simulink library "carnot"  (R2013b)
settings: Solver=ode45  StartTime=0.0  StopTime=10.0  RelTol=1e-3
undefined symbols (not defined in the file or in its folder): A, acol, Ahabit, Awin, Azimuth_Angle, AziWin, B, C, c1, c4, capc, caph, CarnotCallbacks_Density, CarnotCallbacks_Enthalpy, CarnotCallbacks_Enthalpy2Temperature, CarnotCallbacks_Entropy, CarnotCallbacks_Evaporation_Enthalpy, CarnotCallbacks_GlobalMessageLevel, CarnotCallbacks_Grashof, CarnotCallbacks_Heat_Capacity, CarnotCallbacks_Kinematic_Viscosity, CarnotCallbacks_Prandtl, CarnotCallbacks_Saturation_Property, CarnotCallbacks_Saturation_Temperature, CarnotCallbacks_Saturation_Value_Water, CarnotCallbacks_Specific_Volume, CarnotCallbacks_Thermal_Conductivity, CarnotCallbacks_Vapour_Content, CarnotCallbacks_Vapour_Pressure, con, cond, d, Dd, density, dfin, dia, DiameterLastPiece, DPConstant, dpipe, DPLinear, DPQuadratic, emission_out, fluid, FluidMix, FluidType, FPC, frame, g, GeodeticHeight, Gwin, heat_capacity, hgt, HP, Hroom, ID, inlet, K, l, lin, lpipe ... (+29)
undefined symbols (not defined in the file): c2, c3, c5, c6, cwall, dactive, height, mc, mID, rho, tau, UAneighbour, UAwall, uloss
libraries: carnot x333, simulink x25, simulink_extras x7
(part 8 of 16)

== system carnot/Storage/Thermal ==
  Ground_Storage : Subsystem  mask(ground storage){xs=10, ys=10, zs=5, ground=clay (humid), fill=clay (humid), dp=0.1, kp=0.001, zp=1, np=20, t0=20, refine=1, mpts=5}
      mask prompts: xs "extension perpendicular to pipes [m]"; ys "extension parallel to pipes [m]"; zs "depth of storage [m]"; fill "filling"; dp "diameter of pipe [m]"; kp "roughness of pipe [m]"; zp "depth of pipe [m]"; np "number of pipes"; t0 "initial temperature [degree centigrade]"; refine "refine factor"; mpts "number of measurement points"
      mask help:
      | Three-dimensional ground storage model.
      | Look under mask to change the surface model.
      mask init:
      | xs = max(xs, 0.001);
      | ys = max(ys, 0.001);
      | zp = max(zp, 0.001);
      | zs = max(zs, zp);
      | np = max(0, np);
      | dp = max(dp, 0.001);
      | kp = max(kp, 0.001);
      | cond=[0.7 1.88 1.45 2.9 1.28];
      | lg = cond(ground);
      | cap = [1382400 1798200 2410560  2864160 1933800];
      | cg = cap(ground);
      | lf = cond(fill);
      | cf = cap(fill);
      mask Help: web(fullfile(path_carnot('help'),'Ground_Storage.html'),'-helpbrowser')
      mask TypeOptions ground: sand (dry) | sand (saturated with water) | clay (humid) | clay (saturated with water)
      mask TypeOptions fill: sand (dry) | sand (saturated with water) | clay (humid) | clay (saturated with water) | concrete
      mask TypeOptions refine: 1 | 2 | 3 | 4 | 6 | 8 | 10 | 16 | 24 | 32
      mask Display: plot(0,0,100,100,[30,60,70,40,30],[70,70,80,80,70],[68,59,56,59,56,52,48,51,48,44,40,44,41,32],[83,72,72,78,78,72,72,78,78,72,72,78,78,67],[61,58,44,31,30],[69,60,56,60,67],[62,60,52,37,29,29],[68,56,47,48,57,67],[64,67,67,65,57,44,32,27,28],[71,62,53,43,35,35,40,54,66])
  Storage_Ports : Subsystem
      mask Display: plot(0,0,100,100,[10,10,40,40,10],[10,40,40,10,10],[50,70,90,50],[30,65,30,30],[20,10,10,20,30,40,40,30,20],[50,60,70,80,80,70,60,50,50])
  Storage_Type_1 : Subsystem  mask(Multiport Storage){uloss=1, ubot=1, utop=1, cond=1, t0=[10:5:55], volume=0.3, dia=0.5, pos=standing cylinder, nconnect=2, nodes=10, mpoints=10}
      mask prompts: uloss "Heat loss coefficient cylinder wall in W/(m²K)"; ubot "Heat loss coefficient bottom in W/(m²K)"; utop "Heat loss coefficient top cover in W/(m²K)"; cond "Effective vertical conductivity in W/(m*K)"; t0 "Initial temperature (vector or scalar) in °C"; volume "Volume in m³"; dia "Diameter in m"; pos "Position"; nconnect "Number of connections"; nodes "Number of nodes"; mpoints "Number of measurement points"
      mask help:
      | The volmue of the cylindrical storage is divided in a number "nodes" of horizontal slices (1xN-node model). For each node the energy balance equation is solved.
      | Look under mask to set the ports types and properties.
      mask init:
      | [standing, dh, height, mpts, tini] ...
      |     = CarnotCallbacks_StorageTypeN(pos, volume, dia, nodes, mpoints, t0);
      mask Help: web(fullfile(path_carnot('help'),'Storage_Type_N.html'),'-helpbrowser')
      mask TypeOptions pos: lying cylinder | standing cylinder
      mask Display: plot(10,10,90,100,[40,40,45,55,60,60,55,45,40],[84,36,30,30,36,84,90,90,84],[40,35],[77,77],[64,60],[77,77],[40,35],[42,42],[64,60],[42,42])
  Storage_Type_1_CONF : Subsystem  mask(Buffer Storage with 2 connections){parameterfile=default_Storage, tini=[10:5:55]}
      mask prompts: parameterfile "Storage parameter set"; tini "initial temperature (vector or scalar) in °C"
      mask help: Predefinded storage with 2 direct ports (for example a buffer storage tank).
      mask init:
      | % callback to set parameters of model
      | CarnotCallbacks_StorageConf(1,parameterfile);
      mask Help: web(fullfile(path_carnot('help'),'Storage_Type_N.html'),'-helpbrowser')
      mask TypeOptions parameterfile: default_Storage
      mask Display:
      | % user defined picture file
      | picfile = fullfile(path_carnot('intlibsl'), ...
      |     'Storage','Thermal','Storage_Type_1_CONF','parameter_set', ...
      |     'Storage_Type_1_CONF.jpg');
      | 
      | % show public picture
      | plot([40,40,45,55,60,60,55,45,40]/100,[84,36,30,30,36,84,90,90,84]/100, ...
      |     [40,35]/100,[77,77]/100,[64,60]/100,[77,77]/100,[40,35]/100,[42,42]/100, ...
      |     [64,60]/100,[42,42]/100)
      | 
      | % show internal picture if defined
      | if ~BlockIsInCarnotLibrary    % if not located in library any more
      |     if exist(picfile)
      |         image(imread(picfile), [0.3, 0, 0.5, 1])
      |         set_param(gcb, 'BackgroundColor', 'White')
      |     end
      | end
  Storage_Type_2 : Subsystem  mask(Multiport Storage){uloss=1, ubot=1, utop=1, cond=1, t0=[10:5:55], volume=0.3, dia=0.5, pos=standing cylinder, nconnect=2, nodes=10, mpoints=10}
      mask prompts: uloss "Heat loss coefficient cylinder wall in W/(m²K)"; ubot "Heat loss coefficient bottom in W/(m²K)"; utop "Heat loss coefficient top cover in W/(m²K)"; cond "Effective vertical conductivity in W/(m*K)"; t0 "Initial temperature (vector or scalar) in °C"; volume "Volume in m³"; dia "Diameter in m"; pos "Position"; nconnect "Number of connections"; nodes "Number of nodes"; mpoints "Number of measurement points"
      mask help:
      | The volmue of the cylindrical storage is divided in a number "nodes" of horizontal slices (1xN-node model). For each node the energy balance equation is solved.
      | Look under mask to set the ports types and properties.
      mask init:
      | [standing, dh, height, mpts, tini] ...
      |     = CarnotCallbacks_StorageTypeN(pos, volume, dia, nodes, mpoints, t0);
      mask Help: web(fullfile(path_carnot('help'),'Storage_Type_N.html'),'-helpbrowser')
      mask TypeOptions pos: lying cylinder | standing cylinder
      mask Display: plot(10,20,80,100,[36,36,40,50,54,54,50,40,36],[90,50,45,45,50,90,93,93,90],[36,51,44,51,36],[50,50,55,60,60])
  Storage_Type_2_CONF : Subsystem  mask(Storage with 1 heat exchanger and 1 direct port){parameterfile=default_Storage, tini=[10:5:55]}
      mask prompts: parameterfile "Storage parameter set"; tini "initial temperature (vector or scalar) in °C"
      mask help: Predefinded storage with 1 heat exchanger and 1 direct port (for example a dhw cylinder).
      mask init:
      | % callback to set parameters of model
      | CarnotCallbacks_StorageConf(2,parameterfile);
      mask Help: web(fullfile(path_carnot('help'),'Storage_Type_N.html'),'-helpbrowser')
      mask TypeOptions parameterfile: default_Storage
      mask Display:
      | % user defined picture file
      | picfile = fullfile(path_carnot('intlibsl'), ...
      |         'Storage','Thermal','Storage_Type_2_CONF','parameter_set', ...
      |         'Storage_Type_2_CONF.jpg');
      | 
      | % show public picture
      | plot(0.1,0.2,0.80,1,[36,36,40,50,54,54,50,40,36]/100,...
      |     [90,50,45,45,50,90,93,93,90]/100,[36,51,44,51,36]/100,...
      |     [50,50,55,60,60]/100)
      | 
      | % show internal picture if defined
      | if  ~BlockIsInCarnotLibrary       % if not located in library
      |     if exist(picfile)
      |         image(imread(picfile), [0.3, 0, 0.5, 1])
      |         set_param(gcb, 'BackgroundColor', 'White')
      |     end
      | end
  Storage_Type_3 : Subsystem  mask(Multiport Storage){uloss=1, ubot=1, utop=1, cond=1, t0=[10:5:55], volume=0.3, dia=0.5, pos=standing cylinder, nconnect=3, nodes=10, mpoints=10}
      mask prompts: uloss "Heat loss coefficient cylinder wall in W/(m²K)"; ubot "Heat loss coefficient bottom in W/(m²K)"; utop "Heat loss coefficient top cover in W/(m²K)"; cond "Effective (wall and fluid) vertical conductivity in W/(m*K)"; t0 "Initial temperature (vector or scalar) in °C"; volume "Volume in m³"; dia "Diameter in m"; pos "Position"; nconnect "Number of connections"; nodes "Number of nodes"; mpoints "Number of measurement points"
      mask help:
      | The volmue of the cylindrical storage is divided in a number "nodes" of horizontal slices (1xN-node model). For each node the energy balance equation is solved.
      | Look under mask to set the ports types and properties.
      mask init:
      | [standing, dh, height, mpts, tini] ...
      |     = CarnotCallbacks_StorageTypeN(pos, volume, dia, nodes, mpoints, t0);
      mask Help: web(fullfile(path_carnot('help'),'Storage_Type_N.html'),'-helpbrowser')
      mask TypeOptions pos: lying cylinder | standing cylinder
      mask Display: plot(10,20,80,100,[36,36,40,50,54,54,50,40,36],[90,50,45,45,50,90,93,93,90],[36,51,40,51,36],[77,77,81,85,85],[36,51,44,51,36],[50,50,55,60,60])
  Storage_Type_3_CONF : Subsystem  mask(Storage with 2 heat exchangers and 1 direct port){parameterfile=default_Storage, tini=[10:5:55]}
      mask prompts: parameterfile "Storage parameter set"; tini "initial temperature (vector or scalar) in °C"
      mask help: Predefinded storage with 2 heat exchangers and 1 direct port (for example a bivalent dhw cylinder).
      mask init:
      | % callback to set parameters of model
      | CarnotCallbacks_StorageConf(3,parameterfile);
      mask Help: web(fullfile(path_carnot('help'),'Storage_Type_N.html'),'-helpbrowser')
      mask TypeOptions parameterfile: default_Storage
      mask Display:
      | % user defined picture file
      | picfile = fullfile(path_carnot('intlibsl'), ...
      |         'Storage','Thermal','Storage_Type_3_CONF','parameter_set', ...
      |         'Storage_Type_3_CONF.jpg');
      | 
      | % show public picture
      | plot([36,36,40,50,54,54,50,40,36]/100,[90,50,45,45,50,90,93,93,90]/100, ...
      |     [36,51,40,51,36]/100,[77,77,81,85,85]/100,[36,51,44,51,36]/100, ...
      |     [50,50,55,60,60]/100)
      | 
      | % show internal picture if defined
      | if  ~BlockIsInCarnotLibrary       % if not located in library
      |     if exist(picfile)
      |         image(imread(picfile), [0.25, 0, 0.45, 1])
      |         set_param(gcb, 'BackgroundColor', 'White')
      |     end
      | end
  Storage_Type_4 : Subsystem  mask(Multiport Storage){uloss=0.74, ubot=1.37, utop=0.74, cond=0.62, t0=[10:5:55], volume=0.75, dia=0.79, pos=standing cylinder, nconnect=4, nodes=50, mpoints=50}
      mask prompts: uloss "Heat loss coefficient cylinder wall in W/(m²K)"; ubot "Heat loss coefficient bottom in W/(m²K)"; utop "Heat loss coefficient top cover in W/(m²K)"; cond "Effective (wall and fluid) vertical conductivity in W/(m*K)"; t0 "Initial temperature (vector or scalar) in °C"; volume "Volume in m³"; dia "Diameter in m"; pos "Position"; nconnect "Number of connections"; nodes "Number of nodes"; mpoints "Number of measurement points"
      mask help:
      | The volmue of the cylindrical storage is divided in a number "nodes" of horizontal slices (1xN-node model). For each node the energy balance equation is solved.
      | Look under mask to set the ports types and properties.
      mask init:
      | [standing, dh, height, mpts, tini] ...
      |     = CarnotCallbacks_StorageTypeN(pos, volume, dia, nodes, mpoints, t0);
      mask Help: web(fullfile(path_carnot('help'),'Storage_Type_N.html'),'-helpbrowser')
      mask TypeOptions pos: lying cylinder | standing cylinder
      mask Display: plot(5,10,85,110,[36,36,40,50,54,54,50,40,36],[90,50,45,45,50,90,93,93,90],[36,51,40,51,36],[50,50,68,85,85],[36,51,44,51,36],[54,54,56,58,58])
  Storage_Type_4_CONF : Subsystem  mask(Combi-storage for hot water production and heating){parameterfile=Default_Storage, tini=[10:5:55]}
      mask prompts: parameterfile "Storage parameter set"; tini "initial temperature (vector or scalar) in °C"
      mask help: Predefinded combi-storage for hot water production and heating configurated to preheat the return of the backup heater.
      mask init:
      | % callback to set parameters of model
      | CarnotCallbacks_StorageConf(4,parameterfile);
      mask Help: web(fullfile(path_carnot('help'),'Storage_Type_N.html'),'-helpbrowser')
      mask TypeOptions parameterfile: Default_Storage
      mask Display:
      | % user defined picture file
      | picfile = fullfile(path_carnot('intlibsl'), ...
      |         'Storage','Thermal','Storage_Type_4_CONF','parameter_set', ...
      |         'Storage_Type_4_CONF.jpg');
      | 
      | % show public picture
      | plot([36,36,40,50,54,54,50,40,36]/100,[90,50,45,45,50,90,93,93,90]/100, ...
      |     [36,51,40,51,36]/100,[50,50,68,85,85]/100,[36,51,44,51,36]/100, ...
      |     [54,54,56,58,58]/100)
      | 
      | % show internal picture if defined
      | if  ~BlockIsInCarnotLibrary       % if not located in library
      |     if exist(picfile)
      |         image(imread(picfile), [0.3, 0, 0.45, 1])
      |         set_param(gcb, 'BackgroundColor', 'White')
      |     end
      | end
  Storage_Type_5 : Subsystem  mask(Multiport Storage){uloss=0.74, ubot=1.37, utop=0.74, cond=0.62, t0=[10:5:55], volume=0.75, dia=0.79, pos=standing cylinder, nconnect=5, nodes=50, mpoints=50}
      mask prompts: uloss "Heat loss coefficient cylinder wall in W/(m²K)"; ubot "Heat loss coefficient bottom in W/(m²K)"; utop "Heat loss coefficient top cover in W/(m²K)"; cond "Effective (wall and fluid) vertical conductivity in W/(m*K)"; t0 "Initial temperature (vector or scalar) in °C"; volume "Volume in m³"; dia "Diameter in m"; pos "Position"; nconnect "Number of connections"; nodes "Number of nodes"; mpoints "Number of measurement points"
      mask help:
      | The volmue of the cylindrical storage is divided in a number "nodes" of horizontal slices (1xN-node model). For each node the energy balance equation is solved.
      | Look under mask to set the ports types and properties.
      mask init:
      | [standing, dh, height, mpts, tini] ...
      |     = CarnotCallbacks_StorageTypeN(pos, volume, dia, nodes, mpoints, t0);
      mask Help: web(fullfile(path_carnot('help'),'Storage_Type_N.html'),'-helpbrowser')
      mask TypeOptions pos: lying cylinder | standing cylinder
      mask Display: plot(5,10,85,110,[36,36,40,50,54,54,50,40,36],[90,50,45,45,50,90,93,93,90],[36,51,40,51,36],[50,50,68,85,85],[36,51,44,51,36],[54,54,56,58,58])
  Storage_Type_5_CONF : Subsystem  mask(Combi-storage for hot water production and heating){parameterfile=Default_Storage, tini=[10:5:55]}
      mask prompts: parameterfile "Storage parameter set"; tini "initial temperature (vector or scalar) in °C"
      mask help: Predefinded combi-storage for hot water production and heating configurated for parallel buffer operation of the backup heater.
      mask init:
      | % callback to set parameters of model
      | CarnotCallbacks_StorageConf(5,parameterfile);
      mask Help: web(fullfile(path_carnot('help'),'Storage_Type_N.html'),'-helpbrowser')
      mask TypeOptions parameterfile: Default_Storage
      mask Display:
      | % user defined picture file
      | picfile = fullfile(path_carnot('intlibsl'), ...
      |         'Storage','Thermal','Storage_Type_5_CONF','parameter_set', ...
      |         'Storage_Type_5_CONF.jpg');
      | 
      | % show public picture
      | plot([36,36,40,50,54,54,50,40,36]/100,[90,50,45,45,50,90,93,93,90]/100, ...
      |     [36,51,40,51,36]/100,[50,50,68,85,85]/100,[36,51,44,51,36]/100, ...
      |     [54,54,56,58,58]/100)
      | 
      | % show internal picture if defined
      | if  ~BlockIsInCarnotLibrary       % if not located in library
      |     if exist(picfile)
      |         image(imread(picfile), [0.3, 0, 0.45, 1])
      |         set_param(gcb, 'BackgroundColor', 'White')
      |     end
      | end
  detailed_storage_models : Subsystem
      mask Display: plot(0,0,100,100,[10,10,40,40,10],[10,40,40,10,10],[50,70,90,50],[30,65,30,30],[20,10,10,20,30,40,40,30,20],[50,60,70,80,80,70,60,50,50])
  surface_models : Subsystem
      mask Display: plot(0,0,100,100,[10,10,40,40,10],[10,40,40,10,10],[50,70,90,50],[30,65,30,30],[20,10,10,20,30,40,40,30,20],[50,60,70,80,80,70,60,50,50])

== system carnot/Toolbox/Average ==
  input : Inport
  time : Inport  Port=2
  enable : Inport  Port=3
  Demux1 : Demux  Outputs=[-1 1 1]
  Mux : Mux  Inputs=3
  S-Function3 : S-Function  FunctionName=average  Parameters=delta_t offset_flag enable_flag  EnableBusSupport=off
  average : Outport
  output time : Outport  Port=2
  pulse : Outport  Port=3
  wires:
  Mux/1 -> S-Function3/1
  S-Function3/1 -> Demux1/1
  input/1 -> Mux/1
  time/1 -> Mux/2
  enable/1 -> Mux/3
  Demux1/1 -> average/1
  Demux1/2 -> output time/1
  Demux1/3 -> pulse/1

== system carnot/Toolbox/Economy_Ecology ==
  note: mass of fuel in kg
  note: thermal energy in J
  note: electric energy in J
  note: fuel costs
  note: mass of produced H2O
  note: mass of produced CO2
  note: mass of produced O2
  note: mass of produced SO2
  note: mass of produced N2
  note: mass of produced NOx
  note: mass of produced CO
  note: mass of produced CxHy
  eco : Inport
  Count_Working_Time : carnot/Toolbox/Count_Working_Time
  Demux1 : Demux  Outputs=12
  Display : Display
  Integrator : Integrator
  Mux : Mux  Inputs=12
  Mux1 : Mux  Inputs=2
  Selector : Selector  InputPortWidth=19  IndexOptions=Index vector (dialog)  Indices=[3 5:15]  OutputSizes=1
  Selector1 : Selector  InputPortWidth=12  IndexOptions=Index vector (dialog)  Indices=[1]  OutputSizes=1
  Terminator : Terminator
  Terminator1 : Terminator
  Terminator2 : Terminator
  To Workspace : ToWorkspace  VariableName=input_annual_costs  SampleTime=-1
      settings: MaxDataPoints=1
  wires:
  Count_Working_Time/3 -> Terminator2/1
  Count_Working_Time/2 -> Terminator1/1
  Count_Working_Time/1 -> Terminator/1
  Count_Working_Time/4 -> Mux1/2  "Run time"
  Demux1/4 -> Mux1/1, Mux/4  "costs"
  Demux1/1 -> Mux/1  "m_fuel"
  Selector1/1 -> Count_Working_Time/1
  Selector/1 -> Selector1/1, Integrator/1
  Mux1/1 -> To Workspace/1
  Mux/1 -> Display/1
  Demux1/3 -> Mux/3  "E_electric"
  Demux1/2 -> Mux/2  "Qtherm"
  Demux1/10 -> Mux/10  "NOx"
  Demux1/11 -> Mux/11  "CO"
  Demux1/12 -> Mux/12  "CxHy"
  Demux1/9 -> Mux/9  "N2"
  Demux1/6 -> Mux/6  "CO2"
  Integrator/1 -> Demux1/1
  eco/1 -> Selector/1
  Demux1/7 -> Mux/7  "O2"
  Demux1/5 -> Mux/5  "H20"
  Demux1/8 -> Mux/8  "SO2"

== system carnot/Toolbox/GlobalMessageLevel ==

== system carnot/Toolbox/RealDate ==
  Ground : Ground
  S-Function3 : S-Function  FunctionName=systemdate  Parameters=form  EnableBusSupport=off
  date : Outport
  wires:
  S-Function3/1 -> date/1
  Ground/1 -> S-Function3/1

== system carnot/Toolbox/RealTime ==
  Ground : Ground
  S-Function3 : S-Function  FunctionName=systemtime  EnableBusSupport=off
  time : Outport
  wires:
  S-Function3/1 -> time/1
  Ground/1 -> S-Function3/1

== system carnot/Toolbox/RealTimePulse ==
  In : Inport
  S-Function : S-Function  FunctionName=monoflop_realtime  Parameters=time typ  EnableBusSupport=off
  Out : Outport
  wires:
  In/1 -> S-Function/1
  S-Function/1 -> Out/1

== system carnot/Toolbox/SystemPulse ==
  enable pulse : Inport
  Mux : Mux  Inputs=2
  S-Function3 : S-Function  FunctionName=systempulse  Parameters=datecheck enable_flag  EnableBusSupport=off
  position6 : Constant  Value=[date period pulsewidth]
  pulse : Outport
  wires:
  Mux/1 -> S-Function3/1
  enable pulse/1 -> Mux/2
  S-Function3/1 -> pulse/1
  position6/1 -> Mux/1

== system carnot/Toolbox/THB2THV ==
  THB : Inport  OutDataTypeStr=Bus: THB
  Bus Selector : BusSelector  OutputSignals=ID,Temperature,MassFlow,Pressure,FluidType,FluidMix,DiameterLastPiece,DPConstant,DPLinear,DPQuadratic,HydraulicInductance,GeodeticHeight
  Ground : Ground
  Mux : Mux  Inputs=[1 1 1 1 1 1 1 1 1 1 1 1 8]
  THV : Outport
  wires:
  THB/1 -> Bus Selector/1
  Mux/1 -> THV/1
  Bus Selector/1 -> Mux/1  "<ID>"
  Bus Selector/2 -> Mux/2  "<Temperature>"
  Bus Selector/3 -> Mux/3  "<MassFlow>"
  Bus Selector/4 -> Mux/4  "<Pressure>"
  Bus Selector/5 -> Mux/5  "<FluidType>"
  Bus Selector/6 -> Mux/6  "<FluidMix>"
  Bus Selector/7 -> Mux/7  "<DiameterLastPiece>"
  Bus Selector/8 -> Mux/8  "<DPConstant>"
  Bus Selector/9 -> Mux/9  "<DPLinear>"
  Bus Selector/10 -> Mux/10  "<DPQuadratic>"
  Bus Selector/11 -> Mux/11  "<HydraulicInductance>"
  Bus Selector/12 -> Mux/12  "<GeodeticHeight>"
  Ground/1 -> Mux/13

== system carnot/Toolbox/THBMemory ==
  THB_in : Inport  OutDataTypeStr=Bus: THB
  Bus Creator : BusCreator  Inputs=12
  Bus Selector6 : BusSelector  OutputSignals=ID,Temperature,MassFlow,Pressure,FluidType,FluidMix,DiameterLastPiece,DPConstant,DPLinear,DPQuadratic,HydraulicInductance,GeodeticHeight
  Memory_DPConstant : Memory  X0=c
  Memory_DPLinear : Memory  X0=l
  Memory_DPQuadratic : Memory  X0=q
  Memory_DiameterLastPiece : Memory  X0=d
  Memory_FluidMix : Memory  X0=FluidMix
  Memory_FluidType : Memory  X0=FluidType
  Memory_GeodeticHeight : Memory  X0=H
  Memory_HydraulicInductance : Memory  X0=LH
  Memory_ID : Memory  X0=ID
  Memory_MassFlow : Memory  X0=mdot
  Memory_Pressure : Memory  X0=p
  Memory_Temperature : Memory  X0=T
  THB_out : Outport
  wires:
  Bus Selector6/12 -> Memory_GeodeticHeight/1  "<GeodeticHeight>"
  Memory_GeodeticHeight/1 -> Bus Creator/12  "GeodeticHeight"
  Bus Selector6/1 -> Memory_ID/1  "<ID>"
  Memory_ID/1 -> Bus Creator/1  "ID"
  Bus Selector6/2 -> Memory_Temperature/1  "<Temperature>"
  Memory_Temperature/1 -> Bus Creator/2  "Temperature"
  Bus Selector6/3 -> Memory_MassFlow/1  "<MassFlow>"
  Memory_MassFlow/1 -> Bus Creator/3  "MassFlow"
  Bus Selector6/4 -> Memory_Pressure/1  "<Pressure>"
  Memory_Pressure/1 -> Bus Creator/4  "Pressure"
  Bus Selector6/5 -> Memory_FluidType/1  "<FluidType>"
  Memory_FluidType/1 -> Bus Creator/5  "FluidType"
  Bus Selector6/6 -> Memory_FluidMix/1  "<FluidMix>"
  Memory_FluidMix/1 -> Bus Creator/6  "FluidMix"
  Bus Selector6/7 -> Memory_DiameterLastPiece/1  "<DiameterLastPiece>"
  Memory_DiameterLastPiece/1 -> Bus Creator/7  "DiameterLastPiece"
  Bus Selector6/8 -> Memory_DPConstant/1  "<DPConstant>"
  Memory_DPConstant/1 -> Bus Creator/8  "DPConstant"
  Bus Selector6/9 -> Memory_DPLinear/1  "<DPLinear>"
  Memory_DPLinear/1 -> Bus Creator/9  "DPLinear"
  Bus Selector6/10 -> Memory_DPQuadratic/1  "<DPQuadratic>"
  Memory_DPQuadratic/1 -> Bus Creator/10  "DPQuadratic"
  Bus Selector6/11 -> Memory_HydraulicInductance/1  "<HydraulicInductance>"
  Memory_HydraulicInductance/1 -> Bus Creator/11  "HydraulicInductance"
  Bus Creator/1 -> THB_out/1
  THB_in/1 -> Bus Selector6/1

== system carnot/Toolbox/THV2THB ==
  THV : Inport
  Bus Creator : BusCreator  Inputs=12  OutDataTypeStr=Bus: THB
  Demux : Demux  Outputs=[1 1 1 1 1 1 1 1 1 1 1 1 8]
  Terminator : Terminator
  THB : Outport
  wires:
  Demux/13 -> Terminator/1
  Demux/12 -> Bus Creator/12  "GeodeticHeight"
  Demux/10 -> Bus Creator/10  "DPQuadratic"
  Demux/9 -> Bus Creator/9  "DPLinear"
  Demux/8 -> Bus Creator/8  "DPConstant"
  Demux/7 -> Bus Creator/7  "DiameterLastPiece"
  Demux/6 -> Bus Creator/6  "FluidMix"
  Demux/5 -> Bus Creator/5  "FluidType"
  Bus Creator/1 -> THB/1
  Demux/4 -> Bus Creator/4  "Pressure"
  Demux/3 -> Bus Creator/3  "MassFlow"
  Demux/1 -> Bus Creator/1  "ID"
  Demux/2 -> Bus Creator/2  "Temperature"
  THV/1 -> Demux/1
  Demux/11 -> Bus Creator/11  "HydraulicInductance"

== system carnot/Toolbox/UnitConv ==
  In : Inport
  S-Function : S-Function  FunctionName=unitconv_s  Parameters=input_unit output_unit  EnableBusSupport=off
  Out : Outport
  wires:
  In/1 -> S-Function/1
  S-Function/1 -> Out/1

== system carnot/Toolbox/UnitConv_Temperature ==
  Tinit : Inport
  S-Function : S-Function  FunctionName=unitconv_temperature_s  Parameters=ini_unit, fin_unit  EnableBusSupport=off
  Tfinal : Outport
  wires:
  S-Function/1 -> Tfinal/1
  Tinit/1 -> S-Function/1

== system carnot/Toolbox/WDB2Weather ==
  WDB : Inport
  Bus Selector1 : BusSelector  OutputSignals=TimeValueComment,Zenith_Angle,Azimuth_Angle,Solar_Radiation_beam_normal,Solar_Radiation_diffuse_horizontal,Temperature_Ambient,Temperature_Sky_Radiation,Relative_Humidity,Precipitation,Cloud_Index,Station_Pressure,Wind_Speed,Wind_Direction,Incidence_Angle_sun,Incidence_Angle_longitudinal,Incidence_Angle_transversal,Solar_Radiation_direct_surface,Solar_Radiation_diffuse_surface
  Mux : Mux  Inputs=18
  weather : Outport
  wires:
  Bus Selector1/1 -> Mux/1  "<TimeValueComment>"
  Bus Selector1/2 -> Mux/2  "<Zenith_Angle>"
  Bus Selector1/3 -> Mux/3  "<Azimuth_Angle>"
  Bus Selector1/4 -> Mux/4  "<Solar_Radiation_beam_normal>"
  Bus Selector1/5 -> Mux/5  "<Solar_Radiation_diffuse_horizontal>"
  Bus Selector1/6 -> Mux/6  "<Temperature_Ambient>"
  Bus Selector1/7 -> Mux/7  "<Temperature_Sky_Radiation>"
  Bus Selector1/8 -> Mux/8  "<Relative_Humidity>"
  Bus Selector1/9 -> Mux/9  "<Precipitation>"
  Bus Selector1/10 -> Mux/10  "<Cloud_Index>"
  Bus Selector1/11 -> Mux/11  "<Station_Pressure>"
  Bus Selector1/12 -> Mux/12  "<Wind_Speed>"
  Bus Selector1/13 -> Mux/13  "<Wind_Direction>"
  Bus Selector1/14 -> Mux/14  "<Incidence_Angle_sun>"
  Bus Selector1/15 -> Mux/15  "<Incidence_Angle_longitudinal>"
  Bus Selector1/16 -> Mux/16  "<Incidence_Angle_transversal>"
  Bus Selector1/17 -> Mux/17  "<Solar_Radiation_direct_surface>"
  Bus Selector1/18 -> Mux/18  "<Solar_Radiation_diffuse_surface>"
  WDB/1 -> Bus Selector1/1
  Mux/1 -> weather/1

== system carnot/Toolbox/Wait ==
  S-Function3 : S-Function  FunctionName=wait  Parameters=date(1) date(2) date(3) date(4) date(5) wtime  EnableBusSupport=off

== system carnot/Toolbox/Weather2WDB ==
  weather : Inport
  Demux : Demux  Outputs=18
  WDB_Creator : carnot/Basic/Weather_and_Sun/WDB_Creator
  WDB : Outport
  wires:
  weather/1 -> Demux/1
  WDB_Creator/1 -> WDB/1
  Demux/1 -> WDB_Creator/1  "time_value"
  Demux/2 -> WDB_Creator/2  "zenith"
  Demux/3 -> WDB_Creator/3  "azimuth"
  Demux/4 -> WDB_Creator/4  "I_beam_normal"
  Demux/5 -> WDB_Creator/5  "I_diffuse_horizontal"
  Demux/6 -> WDB_Creator/6  "Tamb"
  Demux/7 -> WDB_Creator/7  "Tsky"
  Demux/8 -> WDB_Creator/8  "relative_humidity"
  Demux/9 -> WDB_Creator/9  "precipitation"
  Demux/10 -> WDB_Creator/10  "cloud_index"
  Demux/11 -> WDB_Creator/11  "pressure"
  Demux/12 -> WDB_Creator/12  "wind_speed"
  Demux/13 -> WDB_Creator/13  "wind_direction"
  Demux/14 -> WDB_Creator/14  "incidence_angle"
  Demux/15 -> WDB_Creator/15  "longitudinal_angle"
  Demux/16 -> WDB_Creator/16  "transversal_angle"
  Demux/17 -> WDB_Creator/17  "I_direct_surface"
  Demux/18 -> WDB_Creator/18  "I_diffuse_surface"

== system carnot/Toolbox/write_txt_file ==
  In : Inport
  enable : Inport  Port=2
  Mux1 : Mux  Inputs=2
  S-Function : S-Function  FunctionName=write_txt_file  Parameters=clear filename  EnableBusSupport=off
  Terminator : Terminator
  wires:
  enable/1 -> Mux1/2
  In/1 -> Mux1/1
  Mux1/1 -> S-Function/1
  S-Function/1 -> Terminator/1

== system carnot/Weather/Add_Solar_Position ==
  WDB_in : Inport
  Bus Assignment : BusAssignment  AssignedSignals=Zenith_Angle,Azimuth_Angle
  Demux : Demux  Outputs=2
  Solar_Position : carnot/Basic/Weather_and_Sun/Solar_Position  lati=lati  longi=longi  timezone=timezone
  WDB : Outport
  wires:
  Bus Assignment/1 -> WDB/1
  Demux/2 -> Bus Assignment/3
  Demux/1 -> Bus Assignment/2
  WDB_in/1 -> Bus Assignment/1
  Solar_Position/1 -> Demux/1  "zenith, azimuth"

== system carnot/Weather/DWD_TRY_Radiation_Filter ==
  WDB : Inport
  Bus Assignment : BusAssignment  AssignedSignals=Solar_Radiation_beam_normal,Solar_Radiation_diffuse_horizontal,Solar_Radiation_direct_surface,Solar_Radiation_diffuse_surface
  Bus Selector1 : BusSelector  OutputSignals=Incidence_Angle_sun
  Bus Selector2 : BusSelector  OutputSignals=Solar_Radiation_beam_normal,Solar_Radiation_diffuse_horizontal,Solar_Radiation_direct_surface,Solar_Radiation_diffuse_surface
  Degrees to Radians : simulink_extras/Transformations/Degrees to Radians
  Demux : Demux  Outputs=3
  Gain : Gain  Gain=f
  MinMax : MinMax  Inputs=2
  Mux : Mux  Inputs=3
  Product : Product
  Saturation : Saturate  UpperLimit=inf  LowerLimit=0
  Trigonometric Function : Trigonometry  Operator=cos
  WDB_filter : Outport
  wires:
  Saturation/1 -> MinMax/2
  Gain/1 -> Product/2
  Product/1 -> Saturation/1
  Trigonometric Function/1 -> Gain/1
  Degrees to Radians/1 -> Trigonometric Function/1
  Bus Selector2/1 -> MinMax/1, Product/1  "<Solar_Radiation_beam_normal>"
  Bus Selector2/2 -> Mux/1  "<Solar_Radiation_diffuse_horizontal>"
  MinMax/1 -> Bus Assignment/2  "Solar_Radiation_beam_normal"
  Demux/1 -> Bus Assignment/3  "Solar_Radiation_diffuse_horizontal"
  Demux/3 -> Bus Assignment/5  "Solar_Radiation_diffuse_surface"
  Demux/2 -> Bus Assignment/4  "Solar_Radiation_direct_surface"
  Bus Selector2/4 -> Mux/3  "<Solar_Radiation_diffuse_surface>"
  Bus Selector2/3 -> Mux/2  "<Solar_Radiation_direct_surface>"
  Mux/1 -> Demux/1
  Bus Selector1/1 -> Degrees to Radians/1  "<Incidence_Angle_sun>"
  Bus Assignment/1 -> WDB_filter/1
  WDB/1 -> Bus Assignment/1, Bus Selector1/1, Bus Selector2/1

== system carnot/Weather/Fixed_Surface ==
  Bus Creator : BusCreator  Inputs=3
  collector position : Constant  Value=colangle
  collector position1 : Constant  Value=colazi
  collector position2 : Constant  Value=colrot
  position : Outport
  wires:
  collector position2/1 -> Bus Creator/3  "rotation"
  collector position1/1 -> Bus Creator/2  "azimut"
  collector position/1 -> Bus Creator/1  "inclination"
  Bus Creator/1 -> position/1

== system carnot/Weather/Radiation_on_Inclined_Surface ==
  WDB_in : Inport
  position : Inport  Port=2
  WDB2Weather : carnot/Toolbox/WDB2Weather
  WDB_Creator : carnot/Basic/Weather_and_Sun/WDB_Creator
  radiation_on_surface : S-Function  FunctionName=surfrad  Parameters=sky,reflect  EnableBusSupport=off
  WDB_out : Outport
  wires:
  WDB2Weather/1 -> radiation_on_surface/1
  WDB_Creator/1 -> WDB_out/1
  radiation_on_surface/18 -> WDB_Creator/18  "Solar_Radiation_diffuse_surface"
  radiation_on_surface/17 -> WDB_Creator/17  "Solar_Radiation_direct_surface"
  radiation_on_surface/16 -> WDB_Creator/16  "Incidence_Angle_transversal"
  radiation_on_surface/15 -> WDB_Creator/15  "Incidence_Angle_longitudinal"
  radiation_on_surface/14 -> WDB_Creator/14  "Incidence_Angle_sun"
  radiation_on_surface/13 -> WDB_Creator/13  "Wind_Direction"
  radiation_on_surface/12 -> WDB_Creator/12  "Wind_Speed"
  radiation_on_surface/11 -> WDB_Creator/11  "Station_Pressure"
  radiation_on_surface/10 -> WDB_Creator/10  "Cloud_Index"
  radiation_on_surface/9 -> WDB_Creator/9  "Precipitation"
  radiation_on_surface/8 -> WDB_Creator/8  "Relative_Humidity"
  radiation_on_surface/7 -> WDB_Creator/7  "Temperature_Sky_Radiation"
  radiation_on_surface/6 -> WDB_Creator/6  "Temperature_Ambient"
  radiation_on_surface/5 -> WDB_Creator/5  "Solar_Radiation_diffuse_horizontal"
  radiation_on_surface/4 -> WDB_Creator/4  "Solar_Radiation_beam_normal"
  radiation_on_surface/3 -> WDB_Creator/3  "Azimuth_Angle"
  radiation_on_surface/2 -> WDB_Creator/2  "Zenith_Angle"
  radiation_on_surface/1 -> WDB_Creator/1  "TimeValueComment"
  WDB_in/1 -> WDB2Weather/1
  position/1 -> radiation_on_surface/2

== system carnot/Weather/Select_Weather ==
  weather : Inport
  Selector : Selector  InputPortWidth=18  IndexOptions=Index vector (dialog)  Indices=v  OutputSizes=1
  data : Outport  InitialOutput=0
  wires:
  Selector/1 -> data/1
  weather/1 -> Selector/1

== system carnot/Weather/Tracked_Surface ==
  WDB : Inport
  Bus Creator : BusCreator  Inputs=3
  Bus Selector : BusSelector  OutputSignals=Zenith_Angle,Azimuth_Angle
  Demux : Demux  Outputs=3
  Mux : Mux  Inputs=2
  s-function : S-Function  FunctionName=tracking  Parameters=tracktype time inc azi rot  EnableBusSupport=off
  position : Outport
  wires:
  Bus Selector/2 -> Mux/2  "<Azimuth_Angle>"
  Bus Selector/1 -> Mux/1  "<Zenith_Angle>"
  Mux/1 -> s-function/1
  WDB/1 -> Bus Selector/1
  Demux/1 -> Bus Creator/1  "inclination"
  Demux/2 -> Bus Creator/2  "azimut"
  Demux/3 -> Bus Creator/3  "rotation"
  s-function/1 -> Demux/1
  Bus Creator/1 -> position/1

== system carnot/Weather/WDB2THB ==
  WDB : Inport
  Bus Assignment : BusAssignment  AssignedSignals=Temperature,Pressure,FluidMix
  Bus Selector : BusSelector  OutputSignals=Temperature_Ambient,Relative_Humidity,Station_Pressure
  Constant_THB : carnot/Source/Simple/Constant_THB  t=10  mdot=0  p=1e5  mID=No Pressure Drop  fluid=Air  mix=0  dia=dia  hgt=0
  RelHum2x : carnot/Basic/Material_Properties/RelHum2x
  THB : Outport
  wires:
  RelHum2x/1 -> Bus Assignment/4
  Bus Selector/3 -> Bus Assignment/3, RelHum2x/2  "<Station_Pressure>"
  Bus Selector/2 -> RelHum2x/3  "<Relative_Humidity>"
  Bus Selector/1 -> Bus Assignment/2, RelHum2x/1  "<Temperature_Ambient>"
  Bus Assignment/1 -> THB/1
  Constant_THB/1 -> Bus Assignment/1
  WDB/1 -> Bus Selector/1

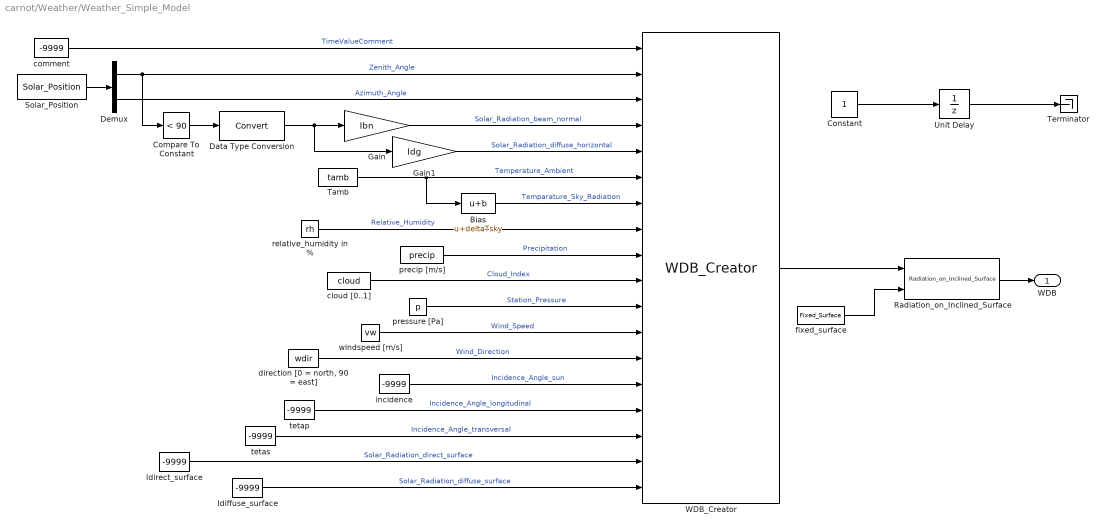
== system carnot/Weather/Weather_Simple_Model ==
  Bias : Bias  Bias=deltaTsky
  Compare To Constant : simulink/Logic and Bit Operations/Compare To Constant  relop=<  const=90  OutDataTypeStr=uint8
  Constant : Constant
  Data Type Conversion : DataTypeConversion
  Demux : Demux  Outputs=2
  Gain : Gain  Gain=Ibn
  Gain1 : Gain  Gain=Idg
  Idiffuse_surface : Constant  Value=-9999
  Idirect_surface : Constant  Value=-9999
  Radiation_on_Inclined_Surface : carnot/Weather/Radiation_on_Inclined_Surface  sky=Perez 1990  reflect=0.2
  Solar_Position : carnot/Basic/Weather_and_Sun/Solar_Position  lati=lat  longi=0  timezone=0
  Tamb : Constant  Value=tamb
  Terminator : Terminator
  Unit Delay : UnitDelay  SampleTime=3600
  WDB_Creator : carnot/Basic/Weather_and_Sun/WDB_Creator
  cloud [0..1] : Constant  Value=cloud
  comment : Constant  Value=-9999
  "direction [0 = north, 90 = east]" : Constant  Value=wdir
  fixed_surface : carnot/Weather/Fixed_Surface  colangle=0  colazi=0  colrot=0
  incidence : Constant  Value=-9999
  precip [m/s] : Constant  Value=precip
  pressure [Pa] : Constant  Value=p
  relative_humidity in % : Constant  Value=rh
  tetap : Constant  Value=-9999
  tetas : Constant  Value=-9999
  windspeed [m/s] : Constant  Value=vw
  WDB : Outport
  wires:
  Unit Delay/1 -> Terminator/1
  Constant/1 -> Unit Delay/1
  Data Type Conversion/1 -> Gain/1, Gain1/1
  Idiffuse_surface/1 -> WDB_Creator/18  "Solar_Radiation_diffuse_surface"
  Idirect_surface/1 -> WDB_Creator/17  "Solar_Radiation_direct_surface"
  tetas/1 -> WDB_Creator/16  "Incidence_Angle_transversal"
  tetap/1 -> WDB_Creator/15  "Incidence_Angle_longitudinal"
  incidence/1 -> WDB_Creator/14  "Incidence_Angle_sun"
  "direction [0 = north, 90 = east]"/1 -> WDB_Creator/13  "Wind_Direction"
  windspeed [m/s]/1 -> WDB_Creator/12  "Wind_Speed"
  pressure [Pa]/1 -> WDB_Creator/11  "Station_Pressure"
  cloud [0..1]/1 -> WDB_Creator/10  "Cloud_Index"
  precip [m/s]/1 -> WDB_Creator/9  "Precipitation"
  relative_humidity in %/1 -> WDB_Creator/8  "Relative_Humidity"
  Bias/1 -> WDB_Creator/7  "Temparature_Sky_Radiation"
  Tamb/1 -> Bias/1, WDB_Creator/6  "Temperature_Ambient"
  Gain1/1 -> WDB_Creator/5  "Solar_Radiation_diffuse_horizontal"
  Compare To Constant/1 -> Data Type Conversion/1
  Demux/2 -> WDB_Creator/3  "Azimuth_Angle"
  Demux/1 -> Compare To Constant/1, WDB_Creator/2  "Zenith_Angle"
  comment/1 -> WDB_Creator/1  "TimeValueComment"
  Solar_Position/1 -> Demux/1
  Gain/1 -> WDB_Creator/4  "Solar_Radiation_beam_normal"
  fixed_surface/1 -> Radiation_on_Inclined_Surface/2
  Radiation_on_Inclined_Surface/1 -> WDB/1
  WDB_Creator/1 -> Radiation_on_Inclined_Surface/1

== system carnot/Weather/Weather_from_File ==
  Constant : Constant
  From_Workspace : FromWorkspace  VariableName=DE_TRY2010_04_averageYear  SampleTime=0  OutputAfterFinalValue=Setting to zero
  Terminator : Terminator
  Unit Delay : UnitDelay  SampleTime=t_sample
  Weather2WDB : carnot/Toolbox/Weather2WDB
  Out1 : Outport
  wires:
  Weather2WDB/1 -> Out1/1
  Unit Delay/1 -> Terminator/1
  Constant/1 -> Unit Delay/1
  From_Workspace/1 -> Weather2WDB/1

== system carnot/Weather/Weather_from_Workspace ==
  Constant : Constant
  From_Workspace : FromWorkspace  VariableName=DE_TRY2010_06_averageYear  SampleTime=0  OutputAfterFinalValue=Setting to zero
  Terminator : Terminator
  Unit Delay : UnitDelay  SampleTime=t_sample
  Weather2WDB : carnot/Toolbox/Weather2WDB
  Out1 : Outport
  wires:
  From_Workspace/1 -> Weather2WDB/1
  Constant/1 -> Unit Delay/1
  Unit Delay/1 -> Terminator/1
  Weather2WDB/1 -> Out1/1

== system carnot/Basic/Hydraulics/Flow_Mixer_basic ==
  THB1 : Inport
  THB2 : Inport  Port=2
  clq : Inport  Port=3
  Bus Assignment : BusAssignment  AssignedSignals=ID,Temperature,MassFlow,Pressure,FluidType,FluidMix,DiameterLastPiece,DPConstant,DPLinear,DPQuadratic
  Bus Selector : BusSelector  OutputSignals=ID
  Bus Selector1 : BusSelector  OutputSignals=ID,DPConstant,DPLinear,DPQuadratic  OutputAsBus=on
  Bus Selector2 : BusSelector  OutputSignals=Pressure  OutputAsBus=on
  Bus Selector3 : BusSelector  OutputSignals=FluidType  OutputAsBus=on
  Bus Selector4 : BusSelector  OutputSignals=DiameterLastPiece  OutputAsBus=on
  Bus Selector6 : BusSelector  OutputSignals=ID
  Bus Selector7 : BusSelector  OutputSignals=ID,DPConstant,DPLinear,DPQuadratic  OutputAsBus=on
  Bus Selector8 : BusSelector  OutputSignals=Pressure  OutputAsBus=on
  Bus Selector9 : BusSelector  OutputSignals=DiameterLastPiece  OutputAsBus=on
  Demux1 : Demux  Outputs=3
  MinMax : MinMax  Function=max  Inputs=2
  MinMax1 : MinMax  Inputs=2
  Mix_T_Mdot : carnot/Basic/Hydraulics/Mix_T_Mdot  mixcalc=Tmix = (mdot1*T1 + mdot2*T2)/(mdot1+mdot2)
  S-Function : S-Function  FunctionName=mix_flow  EnableBusSupport=off
  average_1 : Subsystem
  decrease_ID1 : Subsystem
  decrease_ID2 : Subsystem
  THB : Outport
  ID1 : Outport  Port=2
  ID2 : Outport  Port=3
  fdiv : Outport  Port=4
  wires:
  S-Function/2 -> fdiv/1
  clq/1 -> S-Function/3
  Bus Assignment/1 -> THB/1
  Bus Selector7/1 -> S-Function/2
  Bus Selector2/1 -> MinMax1/1  "p"
  Mix_T_Mdot/2 -> Bus Assignment/4
  Mix_T_Mdot/3 -> Bus Assignment/7
  Mix_T_Mdot/1 -> Bus Assignment/3  "T"
  S-Function/1 -> Demux1/1
  Demux1/3 -> Bus Assignment/11  "qua"
  Demux1/2 -> Bus Assignment/10  "lin"
  Demux1/1 -> Bus Assignment/9  "con"
  Bus Selector1/1 -> S-Function/1
  MinMax1/1 -> Bus Assignment/5  "p"
  average_1/1(Out1) -> Bus Assignment/8
  Bus Selector9/1 -> average_1/2(In2)  "diameter"
  Bus Selector4/1 -> average_1/1(In1)  "diameter"
  Bus Selector8/1 -> MinMax1/2  "p"
  Bus Selector6/1 -> ID2/1, decrease_ID2/1(In1)  "<ID>"
  THB2/1 -> Bus Selector9/1, Bus Selector8/1, Bus Selector6/1, Bus Selector7/1, Mix_T_Mdot/2
  Bus Selector3/1 -> Bus Assignment/6  "fluid"
  MinMax/1 -> Bus Assignment/2  "ID"
  decrease_ID2/1(Out1) -> MinMax/2
  decrease_ID1/1(Out1) -> MinMax/1
  Bus Selector/1 -> ID1/1, decrease_ID1/1(In1)  "<ID>"
  THB1/1 -> Bus Selector4/1, Mix_T_Mdot/1, Bus Selector3/1, Bus Selector2/1, Bus Assignment/1, Bus Selector/1, Bus Selector1/1

== system carnot/Basic/Hydraulics/Grashof ==
  Twall : Inport
  Tinf : Inport  Port=2
  p : Inport  Port=3
  Fluid_Type : Inport  Port=4
  Fluid_Mix : Inport  Port=5
  dimension : Inport  Port=6
  SFunction : S-Function  FunctionName=grashofn  Parameters=DEBUGLEVEL,MAXTOTALMESSAGES,MAXCONSECUTIVEMESSAGES,WRITETOFILE,FILENAME  EnableBusSupport=off
  Gr : Outport
  wires:
  SFunction/1 -> Gr/1
  Fluid_Type/1 -> SFunction/1
  Fluid_Mix/1 -> SFunction/2
  Twall/1 -> SFunction/3
  Tinf/1 -> SFunction/4
  p/1 -> SFunction/5
  dimension/1 -> SFunction/6

== system carnot/Basic/Hydraulics/Mix_T_Mdot ==
  THB1 : Inport
  THB2 : Inport  Port=2
  Add : Sum
  Bus Selector2 : BusSelector  OutputSignals=MassFlow
  Bus Selector3 : BusSelector  OutputSignals=MassFlow
  S-Function : S-Function  FunctionName=mix_temperature  Parameters=mixcalc  EnableBusSupport=off
  select1 : Subsystem
  select2 : Subsystem
  T : Outport
  mdot : Outport  Port=2
  mix : Outport  Port=3
  wires:
  select2/1(Out1) -> S-Function/2
  select1/1(Out1) -> S-Function/1
  S-Function/1 -> T/1  "T"
  THB2/1 -> select2/1(In1), Bus Selector3/1
  S-Function/2 -> mix/1  "mix"
  THB1/1 -> select1/1(In1), Bus Selector2/1
  Bus Selector3/1 -> Add/2  "<MassFlow>"
  Bus Selector2/1 -> Add/1  "<MassFlow>"
  Add/1 -> mdot/1

== system carnot/Basic/Hydraulics/Prandtl ==
  T : Inport
  p : Inport  Port=2
  Fluid_Type : Inport  Port=3
  Fluid_Mix : Inport  Port=4
  SFunction : S-Function  FunctionName=prandtln  Parameters=DEBUGLEVEL,MAXTOTALMESSAGES,MAXCONSECUTIVEMESSAGES,WRITETOFILE,FILENAME  EnableBusSupport=off
  Pr : Outport
  wires:
  SFunction/1 -> Pr/1
  T/1 -> SFunction/3
  p/1 -> SFunction/4
  Fluid_Type/1 -> SFunction/1
  Fluid_Mix/1 -> SFunction/2

== system carnot/Basic/Hydraulics/Pump_basic ==
  THBin : Inport
  control : Inport  Port=2
  Bus Assignment : BusAssignment  AssignedSignals=Temperature,MassFlow
  Bus Selector : BusSelector  OutputSignals=Temperature
  IC : InitialCondition  Value=20
  basic_THB : carnot/Basic/Hydraulics/basic_THB  t=20  mdot=0  p=p0  ID=ID  fluid=fluid_id  mix=mix  dia=dia  hgt=hgt
  electric power : Gain  Gain=power  SaturateOnIntegerOverflow=on  OutDataTypeStr=Inherit: Same as input  ParamDataTypeStr=Inherit: Same as input
  mdot : Gain  Gain=mdotmax  SaturateOnIntegerOverflow=on  OutDataTypeStr=Inherit: Same as input  ParamDataTypeStr=Inherit: Same as input
  THB : Outport
  power : Outport  Port=2
  wires:
  Bus Assignment/1 -> THB/1
  basic_THB/1 -> Bus Assignment/1
  Bus Selector/1 -> IC/1  "<Temperature>"
  THBin/1 -> Bus Selector/1
  electric power/1 -> power/1
  control/1 -> electric power/1, mdot/1
  mdot/1 -> Bus Assignment/3  "mdot"
  IC/1 -> Bus Assignment/2

== system carnot/Basic/Hydraulics/Reynolds ==
  T : Inport
  v : Inport  Port=2
  p : Inport  Port=3
  "fluid, mix" : Inport  Port=4
  dimension : Inport  Port=5
  Demux1 : Demux  Outputs=2
  Kinematic_Viscosity : carnot/Basic/Material_Properties/Kinematic_Viscosity  VariantControl=CarlibClassic  INPUTARGUMENTS=state variables (classic)  DEBUGLEVEL=WARNINGLEVEL  MAXTOTALMESSAGES=inf  MAXCONSECUTIVEMESSAGES=inf  WRITETOFILE=0  FILENAME='errors.txt'
  Product : Product  Inputs=/**  SaturateOnIntegerOverflow=on  InputSameDT=on  OutDataTypeStr=Inherit: Same as first input
  Re : Outport
  wires:
  Product/1 -> Re/1
  v/1 -> Product/2
  dimension/1 -> Product/3
  p/1 -> Kinematic_Viscosity/2
  T/1 -> Kinematic_Viscosity/1
  Demux1/1 -> Kinematic_Viscosity/3
  "fluid, mix"/1 -> Demux1/1
  Kinematic_Viscosity/1 -> Product/1
  Demux1/2 -> Kinematic_Viscosity/4

== system carnot/Basic/Hydraulics/THBCreator ==
  ID : Inport
  Temperature : Inport  Port=2
  MassFlow : Inport  Port=3
  Pressure : Inport  Port=4
  FluidType : Inport  Port=5
  FluidMix : Inport  Port=6
  DiameterLastPiece : Inport  Port=7
  DPConstant : Inport  Port=8
  DPLinear : Inport  Port=9
  DPQuadratic : Inport  Port=10
  HydraulicInductance : Inport  Port=11
  GeodeticHeight : Inport  Port=12
  BusCreator : BusCreator  Inputs=12  OutDataTypeStr=Bus: THB
  THB : Outport
  wires:
  BusCreator/1 -> THB/1
  ID/1 -> BusCreator/1  "ID"
  Temperature/1 -> BusCreator/2  "Temperature"
  MassFlow/1 -> BusCreator/3  "MassFlow"
  Pressure/1 -> BusCreator/4  "Pressure"
  FluidType/1 -> BusCreator/5  "FluidType"
  FluidMix/1 -> BusCreator/6  "FluidMix"
  DiameterLastPiece/1 -> BusCreator/7  "DiameterLastPiece"
  DPConstant/1 -> BusCreator/8  "DPConstant"
  DPLinear/1 -> BusCreator/9  "DPLinear"
  DPQuadratic/1 -> BusCreator/10  "DPQuadratic"
  HydraulicInductance/1 -> BusCreator/11  "HydraulicInductance"
  GeodeticHeight/1 -> BusCreator/12  "GeodeticHeight"

== system carnot/Basic/Hydraulics/Velocity ==
  T : Inport
  mdot : Inport  Port=2
  p : Inport  Port=3
  "fluid, mix" : Inport  Port=4
  d : Inport  Port=5
  Demux1 : Demux  Outputs=2
  Density : carnot/Basic/Material_Properties/Density  VariantControl=CarlibClassic  INPUTARGUMENTS=state variables (classic)  DEBUGLEVEL=DEBUGLEVEL  MAXTOTALWARNINGS=inf  MAXCONSECUTIVEWARNINGS=inf  WRITETOFILE=0  FILENAME='errors.txt'
  Math Function : Math  Operator=square  SaturateOnIntegerOverflow=on
  Product : Product  Inputs=*//  SaturateOnIntegerOverflow=on  InputSameDT=on  OutDataTypeStr=Inherit: Same as first input
  quadratic : Gain  Gain=pi/4  SaturateOnIntegerOverflow=on  OutDataTypeStr=Inherit: Same as input  ParamDataTypeStr=Inherit: Same as input
  v : Outport
  density : Outport  Port=2
  wires:
  p/1 -> Density/2
  "fluid, mix"/1 -> Demux1/1
  Demux1/1 -> Density/3
  mdot/1 -> Product/1
  Demux1/2 -> Density/4
  T/1 -> Density/1
  Product/1 -> v/1
  d/1 -> Math Function/1
  Math Function/1 -> quadratic/1
  quadratic/1 -> Product/2
  Density/1 -> Product/3, density/1

== system carnot/Basic/Hydraulics/basic_THB ==
  Bus Creator : BusCreator  InitFcn=load THB.mat  Inputs=12  OutDataTypeStr=Bus: THB
  const{1,22..23,30..31} (5 alike) : Constant  Value=0
  const21 : Constant  Value=ID
  const24 : Constant  Value=t
  const25 : Constant  Value=mdot
  const26 : Constant  Value=p
  const27 : Constant  Value=fluid
  const28 : Constant  Value=mix
  const29 : Constant  Value=dia
  THB : Outport
  wires:
  const30/1 -> Bus Creator/8  "DPConstant"
  const29/1 -> Bus Creator/7  "DiameterLastPiece"
  const28/1 -> Bus Creator/6  "FluidMix"
  const27/1 -> Bus Creator/5  "FluidType"
  const26/1 -> Bus Creator/4  "Pressure"
  const25/1 -> Bus Creator/3  "MassFlow"
  const24/1 -> Bus Creator/2  "Temperature"
  const21/1 -> Bus Creator/1  "ID"
  Bus Creator/1 -> THB/1
  const22/1 -> Bus Creator/9  "DPLinear"
  const23/1 -> Bus Creator/10  "DPQuadratic"
  const31/1 -> Bus Creator/11  "HydraulicInductance"
  const1/1 -> Bus Creator/12  "GeodeticHeight"

== system carnot/Basic/Hydraulics/basic_create_THB ==
  mdot : Inport
  T : Inport  Port=2
  THB_set_T : carnot/Source/Simple/THB_set_T
  THB_set_mdot : carnot/Source/Simple/THB_set_mdot
  basic_THB : carnot/Basic/Hydraulics/basic_THB  t=10  mdot=0  p=p  ID=1  fluid=fluid  mix=mix  dia=dia  hgt=hgt
  THB : Outport
  wires:
  T/1 -> THB_set_T/2
  THB_set_T/1 -> THB/1
  THB_set_mdot/1 -> THB_set_T/1
  mdot/1 -> THB_set_mdot/2
  basic_THB/1 -> THB_set_mdot/1

== system carnot/Basic/Material_Properties/AIV_WetBulbTemperature ==
  AIV : Inport
  AIV_selector : carnot/Outputs/AIV_selector  e1=off  e2=on  e3=off  e4=off  e5=off  e6=off  e7=off  e8=off  e9=off
  AIV_selector1 : carnot/Outputs/AIV_selector  e1=off  e2=off  e3=off  e4=off  e5=off  e6=off  e7=off  e8=on  e9=off
  AIV_selector2 : carnot/Outputs/AIV_selector  e1=off  e2=off  e3=off  e4=on  e5=off  e6=off  e7=off  e8=off  e9=off
  Bus Assignment : BusAssignment  AssignedSignals=Temperature,Pressure,FluidMix
  Constant_THB : carnot/Source/Simple/Constant_THB  t=20  mdot=0  p=1e5  mID=No Pressure Drop  fluid=Air  mix=0  dia=0.02  hgt=0
  THB_WetBulbTemperature : carnot/Basic/Material_Properties/THB_WetBulbTemperature
  WBT : Outport
  rel_hum : Outport  Port=2
  wires:
  THB_WetBulbTemperature/2 -> rel_hum/1
  Bus Assignment/1 -> THB_WetBulbTemperature/1
  Constant_THB/1 -> Bus Assignment/1
  AIV_selector1/1 -> Bus Assignment/3  "p"
  AIV_selector2/1 -> Bus Assignment/4  "mix"
  AIV_selector/1 -> Bus Assignment/2  "T"
  AIV/1 -> AIV_selector/1, AIV_selector2/1, AIV_selector1/1
  THB_WetBulbTemperature/1 -> WBT/1

== system carnot/Basic/Material_Properties/Density ==
  T : Inport
  p : Inport  Port=2
  Fluid_Type : Inport  Port=3
  Fluid_Mix : Inport  Port=4
  SFunction : S-Function  FunctionName=rhofluid  Parameters=DEBUGLEVEL-1,MAXTOTALWARNINGS,MAXCONSECUTIVEWARNINGS,WRITETOFILE,FILENAME  EnableBusSupport=off
  density : Outport
  wires:
  SFunction/1 -> density/1
  T/1 -> SFunction/3
  p/1 -> SFunction/4
  Fluid_Type/1 -> SFunction/1
  Fluid_Mix/1 -> SFunction/2

== system carnot/Basic/Material_Properties/Enthalpy ==
  T : Inport
  p : Inport  Port=2
  Fluid_Type : Inport  Port=3
  Fluid_Mix : Inport  Port=4
  SFunction : S-Function  FunctionName=enthaflu  Parameters=DEBUGLEVEL,MAXTOTALMESSAGES,MAXCONSECUTIVEMESSAGES,WRITETOFILE,FILENAME  EnableBusSupport=off
  enthalpy : Outport
  wires:
  SFunction/1 -> enthalpy/1
  T/1 -> SFunction/3
  p/1 -> SFunction/4
  Fluid_Type/1 -> SFunction/1
  Fluid_Mix/1 -> SFunction/2

== system carnot/Basic/Material_Properties/Enthalpy2Temperature ==
  enthalpy : Inport
  p : Inport  Port=2
  Fluid_Type : Inport  Port=3
  Fluid_Mix : Inport  Port=4
  SFunction : S-Function  FunctionName=enth2temp  Parameters=DEBUGLEVEL,MAXTOTALMESSAGES,MAXCONSECUTIVEMESSAGES,WRITETOFILE,FILENAME  EnableBusSupport=off
  T : Outport
  wires:
  SFunction/1 -> T/1
  Fluid_Type/1 -> SFunction/1
  Fluid_Mix/1 -> SFunction/2
  enthalpy/1 -> SFunction/3
  p/1 -> SFunction/4
